simulink model "vazba"  (Simulink 7.5)
settings: Solver=ode45  StartTime=0.0  StopTime=10.0  RelTol=1e-3
settings Model: Creator=michal  LastModifiedBy=michal

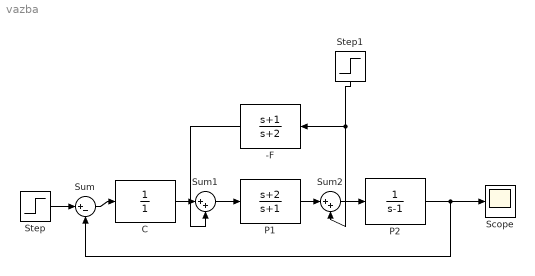
== system vazba ==
  -F : TransferFcn  Numerator=[1 1]  Denominator=[1 2]
  C : TransferFcn  Denominator=[1]
  P1 : TransferFcn  Numerator=[1 2]  Denominator=[1 1]
  P2 : TransferFcn  Denominator=[1 -1]
  Scope : Scope
  Step : Step  SampleTime=0
  Step1 : Step  Time=5  SampleTime=0
  Sum : Sum  Inputs=|+-  OutDataType=fixdt(1, 16)  OutScaling=2^0
  Sum1 : Sum  Inputs=|++  OutDataType=fixdt(1, 16)  OutScaling=2^0
  Sum2 : Sum  Inputs=|++  OutDataType=fixdt(1, 16)  OutScaling=2^0
  wires:
  Sum/1 -> C/1
  Step/1 -> Sum/1
  P2/1 -> Scope/1, Sum/2
  Sum2/1 -> P2/1
  P1/1 -> Sum2/1
  Sum1/1 -> P1/1
  Step1/1 -> -F/1, Sum2/2
  -F/1 -> Sum1/2
  C/1 -> Sum1/1
